simulink model "Zustandsregler"  (Simulink 8.7)
settings: Solver=VariableStepAuto  StartTime=0.0  StopTime=10.0  RelTol=1e-3
values from neighbouring files (symbols this model uses):
  K = R(1:end-1)    [zustandsregler.m]
  Ki = -R(end)    [zustandsregler.m]
  L = H*P    [reglerentwurf.m]    (also in systemidentifikation.m = length(noise_in.Time); zustandsregler.m = acker(A', C', p_b)')
undefined symbols (not defined in the file or in its folder): A, B, C
settings Model: Creator=Oliver  LastModifiedBy=Oliver
settings DataIOCC: LimitDataPoints=off  SaveFormat=Dataset
settings DebuggingCC: UnderspecifiedInitializationDetection=Simplified  MergeDetectMultiDrivingBlocksExec=error
settings HardwareCC: ProdBitPerPointer=64  ProdLargestAtomicFloat=Float  ProdIntDivRoundTo=Zero  ProdEndianess=LittleEndian  ProdWordSize=64  ProdHWDeviceType=Intel->x86-64 (Windows64)
settings ModelReferenceCC: PropagateSignalLabelsOutOfModel=on
settings ConfigComp: CovModelRefEnable=off

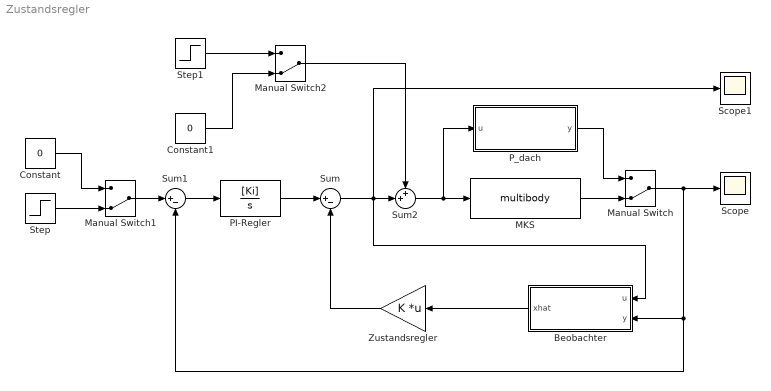
== system Zustandsregler ==
  Beobachter : Subsystem
  Constant : Constant  Value=0
  Constant1 : Constant  Value=0
  MKS : S-Function  FunctionName=multibody  Parameters='Kiethe'  SFunctionDeploymentMode=off  EnableBusSupport=off
  Manual Switch : ManualSwitch  CurrentSetting=0
  Manual Switch1 : ManualSwitch  CurrentSetting=0
  Manual Switch2 : ManualSwitch  CurrentSetting=0
  PI-Regler : TransferFcn  Numerator=[Ki]  Denominator=[1 0]
  P_dach : Subsystem
  Scope : Scope
  Scope1 : Scope
  Step : Step  Time=0  SampleTime=0
  Step1 : Step  SampleTime=0
  Sum : Sum  Inputs=|+-
  Sum1 : Sum  Inputs=|+-
  Sum2 : Sum  Inputs=++|
  Zustandsregler : Gain  Gain=K  Multiplication=Matrix(K*u)
  wires:
  Beobachter/1(xhat) -> Zustandsregler/1
  MKS/1 -> Manual Switch/2
  P_dach/1(y) -> Manual Switch/1
  Manual Switch/1 -> Scope/1, Sum1/2, Beobachter/2(y)
  Sum1/1 -> PI-Regler/1
  Sum/1 -> Sum2/2, Beobachter/1(u), Scope1/1
  PI-Regler/1 -> Sum/1
  Zustandsregler/1 -> Sum/2
  Sum2/1 -> P_dach/1(u), MKS/1
  Manual Switch1/1 -> Sum1/1
  Step/1 -> Manual Switch1/2
  Constant/1 -> Manual Switch1/1
  Manual Switch2/1 -> Sum2/1
  Step1/1 -> Manual Switch2/1
  Constant1/1 -> Manual Switch2/2

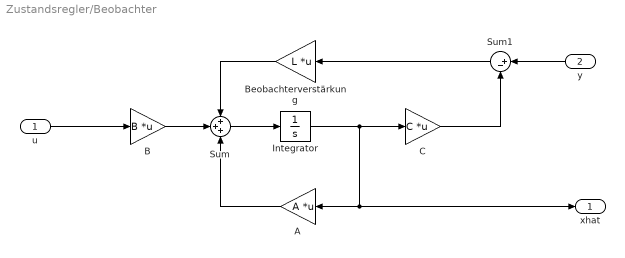
== system Zustandsregler/Beobachter ==
  u : Inport
  y : Inport  Port=2
  A : Gain  Gain=A  Multiplication=Matrix(K*u)
  B : Gain  Gain=B  Multiplication=Matrix(K*u)
  Beobachterverstärkung : Gain  Gain=L  Multiplication=Matrix(K*u)
  C : Gain  Gain=C  Multiplication=Matrix(K*u)
  Integrator : Integrator
  Sum : Sum  Inputs=+++
  Sum1 : Sum  Inputs=|+-
  xhat : Outport
  wires:
  y/1 -> Sum1/1
  C/1 -> Sum1/2
  Sum1/1 -> Beobachterverstärkung/1
  Beobachterverstärkung/1 -> Sum/1
  B/1 -> Sum/2
  A/1 -> Sum/3
  Sum/1 -> Integrator/1
  Integrator/1 -> xhat/1, A/1, C/1
  u/1 -> B/1

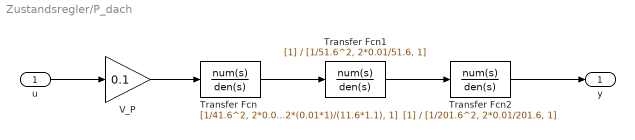
== system Zustandsregler/P_dach ==
  u : Inport
  Transfer Fcn : TransferFcn  Numerator=[1/41.6^2, 2*0.01/41.6, 1]  Denominator=[1/(11.6*1.1)^2, 2*(0.01*1)/(11.6*1.1), 1]
  Transfer Fcn1 : TransferFcn  Denominator=[1/51.6^2, 2*0.01/51.6, 1]
  Transfer Fcn2 : TransferFcn  Denominator=[1/201.6^2, 2*0.01/201.6, 1]
  V_P : Gain  Gain=0.1
  y : Outport
  wires:
  u/1 -> V_P/1
  V_P/1 -> Transfer Fcn/1
  Transfer Fcn/1 -> Transfer Fcn1/1
  Transfer Fcn1/1 -> Transfer Fcn2/1
  Transfer Fcn2/1 -> y/1
